simulink model "localization"  (R2025a)
settings: Solver=ode1  StartTime=0.0  StopTime=Inf  FixedStep=0.2  RelTol=1e-3
PostLoadFcn:
  | qlabs_setup
model workspace (MAT data in the model file):
  mainStepSize = Simulink.Parameter
  mainStepSize.Value = Simulink.data.Expression
  mainStepSize.Value.ExpressionString = "qc_get_step_size"
  mainStepSize.Complexity = 'real'
  mainStepSize.Dimensions = -1
  mainStepSize.DataType = 'auto'
  mode = Simulink.Parameter
  mode.Value = 1
  mode.Complexity = 'real'
  mode.Dimensions = [1 1]
  mode.Description = '0 - education speeds via wheel speed commands
    | 1 - education speeds via body speed commands
    | 2 - research speeds via wheel speed commands
    | 3 - research speeds via body speed commands'
  mode.DataType = 'auto'
  realSenseStepSize = Simulink.Parameter
  realSenseStepSize.Value = Simulink.data.Expression
  realSenseStepSize.Value.ExpressionString = "qc_get_step_size*ceil(1/30/qc_get_step_size)"
  realSenseStepSize.Complexity = 'real'
  realSenseStepSize.Dimensions = -1
  realSenseStepSize.DataType = 'auto'
undefined symbols (not defined in the file): Point
libraries: quarc_library x17, simulink x1
settings Model: SimulationMode=external  ExtModeTrigDuration=10000  Creator=mbohra  LastModifiedBy=rdu
settings DebuggingCC: UnderspecifiedInitializationDetection=Classic  MergeDetectMultiDrivingBlocksExec=none
settings ModelReferenceCC: PropagateSignalLabelsOutOfModel=off
settings RTWCC: GPUComputeCapability=3.5

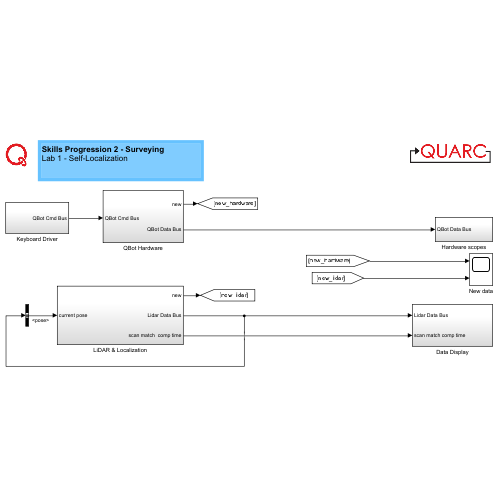
[thumbnail: Simulink's stored preview of the top-level diagram]
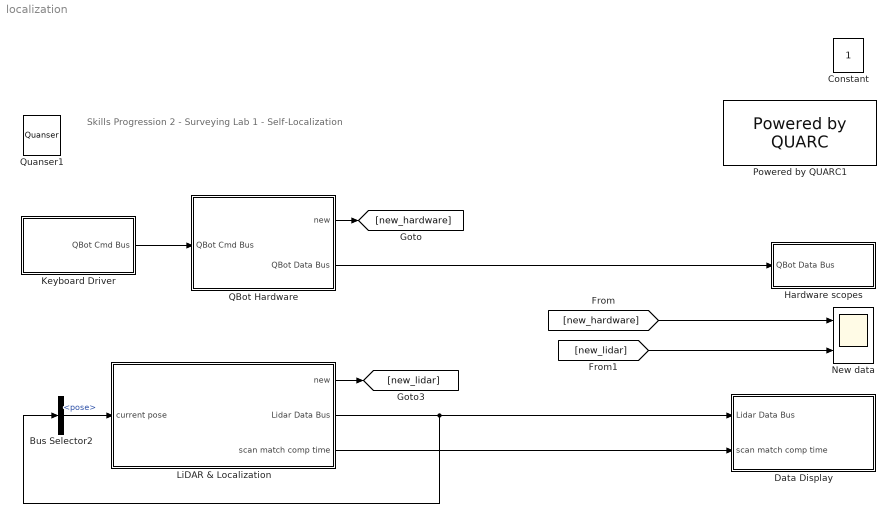
== system localization ==
  note: Skills Progression 2 - Surveying
      | Lab 1 - Self-Localization
  Bus Selector2 : BusSelector  OutputSignals=pose
  Data Display : Subsystem
  Hardware scopes : Subsystem
  Keyboard Driver : Subsystem
  LiDAR & Localization : Subsystem
  New data : Scope  NumInputPorts=2
      settings: Title=Lidar Data New?  ActiveDisplayYMinimum=0.9  ActiveDisplayYMaximum=1.1  DataLoggingVariableName=ScopeData2
  Powered by QUARC1 : quarc_library/Logos/Powered by QUARC
  QBot Hardware : Subsystem
  Quanser1 : quarc_library/Logos/Quanser
  Constant : Constant  IOType=siggen  VectorParams1D=off  SampleTime=1
  wires:
  QBot Hardware/2(QBot Data Bus) -> Hardware scopes/1(QBot Data Bus)
  QBot Hardware/1(new) -> [new_hardware]
  LiDAR & Localization/1(new) -> [new_lidar]
  [new_lidar] -> New data/2
  [new_hardware] -> New data/1
  LiDAR & Localization/2(Lidar Data Bus) -> Data Display/1(Lidar Data Bus), Bus Selector2/1
  Bus Selector2/1 -> LiDAR & Localization/1(current pose)  "<pose>"
  LiDAR & Localization/3(scan match comp time) -> Data Display/2(scan match comp time)
  Keyboard Driver/1(QBot Cmd Bus) -> QBot Hardware/1(QBot Cmd Bus)

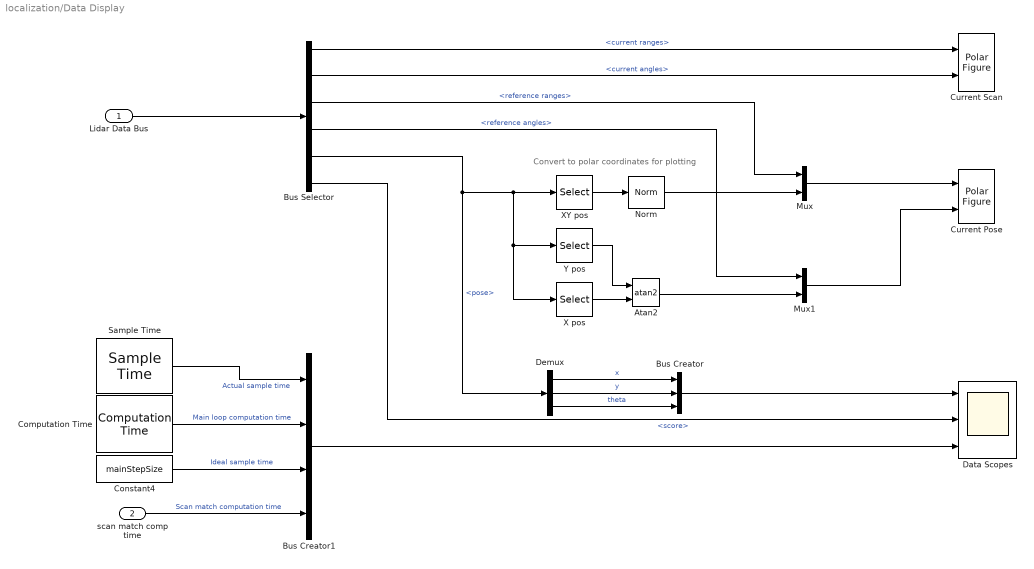
== system localization/Data Display ==
  note: Convert to polar coordinates for plotting
  Lidar Data Bus : Inport
  scan match comp time : Inport  Port=2
  Atan2 : Trigonometry  Operator=atan2
  Bus Creator : BusCreator  Inputs=3
  Bus Creator1 : BusCreator  Inputs=4
  Bus Selector : BusSelector  OutputSignals=current ranges,current angles,reference ranges,reference angles,pose,score
  Computation Time : quarc_library/Sources/Time/Computation Time  sample_time=mainStepSize  use_model=on  use_cpu_time=off
  Constant4 : Constant  Value=mainStepSize
  Current Pose : quarc_library/Sinks/Figures/Polar Figure  figure_mode=Use figure window  figure_tag=figure1  axes_tag=axes1  plot_mode=Time-based  minimum_rho=0  maximum_rho=2  minimum_theta=0  maximum_theta=360  zero_location=right  direction=counterclockwise  buffer_size=2  update_rate=1  sample_time=-1  initial_position="-1516   -95  1081   654"  initial_visibility=off  line1_style=None  line1_width=0.5  line1_color=[1 0 0]  marker1=Point (.)  marker1_size=6  marker1_edge_color=[1 0 0]  marker1_face_color=[1 0 0]  line2_style=Solid line (-)  line2_width=0.5  line2_color=[0.85098 0.32549 0.0980392]  marker2=None  marker2_size=6  marker2_edge_color=[0.85098 0.32549 0.0980392]  marker2_face_color=[0.85098 0.32549 0.0980392]  line3_style=Solid line (-)  line3_width=0.5  line3_color=[0.929412 0.694118 0.12549]  marker3=None  marker3_size=6  marker3_edge_color=[0.929412 0.694118 0.12549]  marker3_face_color=[0.929412 0.694118 0.12549]  line4_style=Solid line (-)  line4_width=0.5  line4_color=[0.494118 0.184314 0.556863]  marker4=None  marker4_size=6  marker4_edge_color=[0.494118 0.184314 0.556863]  marker4_face_color=[0.494118 0.184314 0.556863]  line5_style=Solid line (-)  line5_width=0.5  line5_color=[0.466667 0.67451 0.188235]  marker5=None  marker5_size=6  marker5_edge_color=[0.466667 0.67451 0.188235]  marker5_face_color=[0.466667 0.67451 0.188235]
      settings: SourceProductName=QUARC Targets
  Current Scan : quarc_library/Sinks/Figures/Polar Figure  figure_mode=Use figure window  figure_tag=figure1  axes_tag=axes1  plot_mode=Time-based  minimum_rho=0  maximum_rho=4  minimum_theta=0  maximum_theta=360  zero_location=right  direction=counterclockwise  buffer_size=2  update_rate=1  sample_time=-1  initial_position="370  243  940  693"  initial_visibility=off  line1_style=None  line1_width=0.5  line1_color=[1 0 0]  marker1=Point (.)  marker1_size=6  marker1_edge_color=[1 0 0]  marker1_face_color=[1 0 0]  line2_style=Solid line (-)  line2_width=0.5  line2_color=[0.85098 0.32549 0.0980392]  marker2=None  marker2_size=6  marker2_edge_color=[0.85098 0.32549 0.0980392]  marker2_face_color=[0.85098 0.32549 0.0980392]  line3_style=Solid line (-)  line3_width=0.5  line3_color=[0.929412 0.694118 0.12549]  marker3=None  marker3_size=6  marker3_edge_color=[0.929412 0.694118 0.12549]  marker3_face_color=[0.929412 0.694118 0.12549]  line4_style=Solid line (-)  line4_width=0.5  line4_color=[0.494118 0.184314 0.556863]  marker4=None  marker4_size=6  marker4_edge_color=[0.494118 0.184314 0.556863]  marker4_face_color=[0.494118 0.184314 0.556863]  line5_style=Solid line (-)  line5_width=0.5  line5_color=[0.466667 0.67451 0.188235]  marker5=None  marker5_size=6  marker5_edge_color=[0.466667 0.67451 0.188235]  marker5_face_color=[0.466667 0.67451 0.188235]
      settings: SourceProductName=QUARC Targets
  Data Scopes : Scope  NumInputPorts=3
      settings: ActiveDisplayString=3  Title=Timing  ActiveDisplayYMinimum=-0.051018299999999989  ActiveDisplayYMaximum=0.45916470000000004
  Demux : Demux  Outputs=3
  Mux : Mux  Inputs=2
  Mux1 : Mux  Inputs=2
  Norm : quarc_library/Math Operations/Vectors/Norm
      settings: SourceProductName=QUARC Targets
  Sample Time : quarc_library/Sources/Time/Sample Time  Priority=-99  sample_time=mainStepSize
  X pos : Selector  InputPortWidth=3  IndexOptions=Index vector (dialog)  Indices=[1]  OutputSizes=1
  "XY pos " : Selector  InputPortWidth=3  IndexOptions=Index vector (dialog)  Indices=[1 2]  OutputSizes=1
  Y pos : Selector  InputPortWidth=3  IndexOptions=Index vector (dialog)  Indices=2  OutputSizes=1
  wires:
  Demux/3 -> Bus Creator/3  "theta"
  Demux/2 -> Bus Creator/2  "y"
  Demux/1 -> Bus Creator/1  "x"
  Bus Creator/1 -> Data Scopes/1
  Bus Selector/6 -> Data Scopes/2  "<score>"
  Sample Time/1 -> Bus Creator1/1  "Actual sample time"
  Computation Time/1 -> Bus Creator1/2  "Main loop computation time"
  Constant4/1 -> Bus Creator1/3  "Ideal sample time"
  Bus Creator1/1 -> Data Scopes/3
  scan match comp time/1 -> Bus Creator1/4  "Scan match computation time"
  Bus Selector/2 -> Current Scan/2  "<current angles>"
  Y pos/1 -> Atan2/1
  Bus Selector/3 -> Mux/1  "<reference ranges>"
  Bus Selector/4 -> Mux1/1  "<reference angles>"
  Bus Selector/1 -> Current Scan/1  "<current ranges>"
  Atan2/1 -> Mux1/2
  Bus Selector/5 -> Demux/1, X pos/1, Y pos/1, "XY pos "/1  "<pose>"
  Norm/1 -> Mux/2
  X pos/1 -> Atan2/2
  "XY pos "/1 -> Norm/1
  Lidar Data Bus/1 -> Bus Selector/1
  Mux/1 -> Current Pose/1
  Mux1/1 -> Current Pose/2

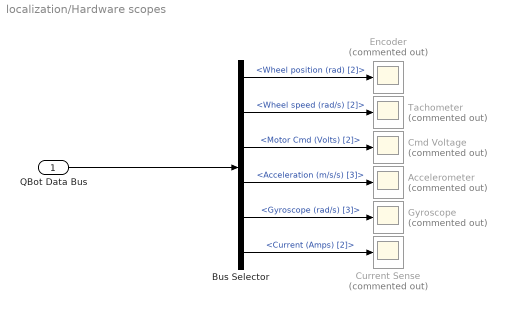
== system localization/Hardware scopes ==
  QBot Data Bus : Inport
  Accelerometer : Scope  Commented=on
      settings: ActiveDisplayYMinimum=-1.32758  ActiveDisplayYMaximum=11.23  DataLoggingVariableName=ScopeData5
  Bus Selector : BusSelector  OutputSignals=Wheel position (rad) [2],Wheel speed (rad/s) [2],Motor Cmd (Volts) [2],Acceleration (m/s/s) [3],Gyroscope (rad/s) [3],Current (Amps) [2]
  Cmd Voltage : Scope  Commented=on
      settings: ActiveDisplayYMinimum=-1  ActiveDisplayYMaximum=1  DataLoggingVariableName=ScopeData4
  Current Sense : Scope  Commented=on
      settings: ActiveDisplayYMinimum=-0.05029  ActiveDisplayYMaximum=0.45265  DataLoggingVariableName=ScopeData7
  Encoder : Scope  Commented=on
      settings: ActiveDisplayYMinimum=-23.46955  ActiveDisplayYMaximum=23.65434  DataLoggingVariableName=ScopeData8
  Gyroscope : Scope  Commented=on
      settings: ActiveDisplayYMinimum=-0.40322  ActiveDisplayYMaximum=1.99912  DataLoggingVariableName=ScopeData6
  Tachometer : Scope  Commented=on
      settings: ActiveDisplayYMinimum=-11.69986  ActiveDisplayYMaximum=11.67552  DataLoggingVariableName=ScopeData3
  wires:
  Bus Selector/2 -> Tachometer/1  "<Wheel speed (rad/s) [2]>"
  Bus Selector/6 -> Current Sense/1  "<Current (Amps) [2]>"
  Bus Selector/3 -> Cmd Voltage/1  "<Motor Cmd (Volts) [2]>"
  Bus Selector/4 -> Accelerometer/1  "<Acceleration (m/s/s) [3]>"
  Bus Selector/5 -> Gyroscope/1  "<Gyroscope (rad/s) [3]>"
  Bus Selector/1 -> Encoder/1  "<Wheel position (rad) [2]>"
  QBot Data Bus/1 -> Bus Selector/1

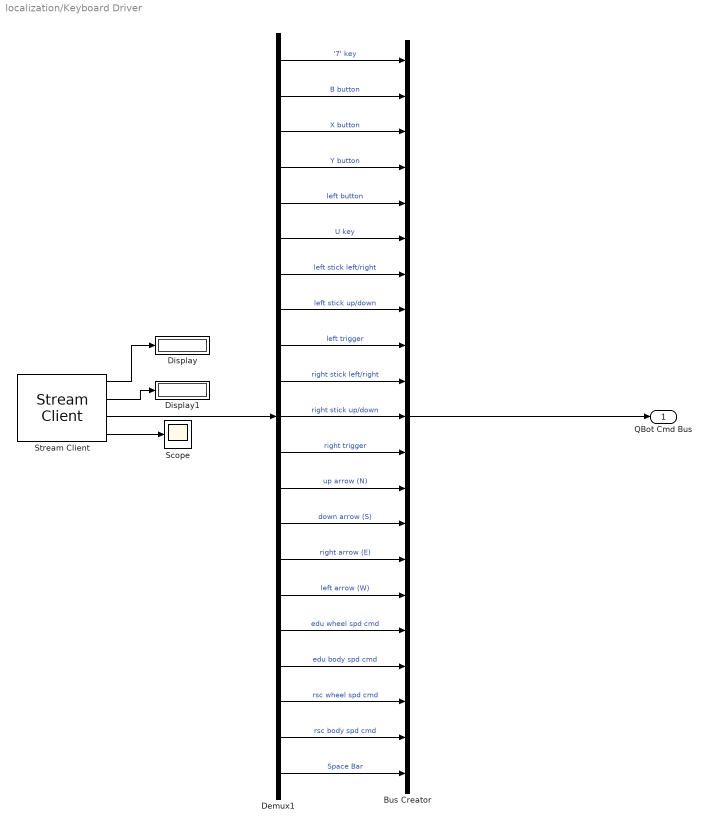
== system localization/Keyboard Driver ==
  Bus Creator : BusCreator  Inputs=21
  Demux1 : Demux  Outputs=[1 1 1 1 1 1 1 1 1 1 1 1 1 1 1 1 2 2 2 2 1]
  Display : Display
  Display1 : Display
  Scope : Scope
      settings: ActiveDisplayYMinimum=-0.125  ActiveDisplayYMaximum=1.125
  Stream Client : quarc_library/Communications/Basic/Stream Client  uri_source=Specify via dialog (do not evaluate)  uri=tcpip://localhost:18889?nagle='off'  send_buffer_size=1460  receive_buffer_size=1460  byte_order=little endian (Intel - LSB first)  optimization=Minimum latency  send_options=Do not send data  receive_options=Receive most recent data  default_value=zeros(25,1)  sample_time=mainStepSize  active=on  implementation=Use blocking I/O in a separate thread  send_fifo_size=1000  receive_fifo_size=1000  send_priority=0  receive_priority=0  send_dimensions=off  receive_dimensions=off  max_dimensions=-1  data_type=Inherited via back propagation  type_expr=BusObject
      settings: AttributesFormatString="\"tcpip://localhost:18889?nagle='off'\""
  QBot Cmd Bus : Outport
  wires:
  Bus Creator/1 -> QBot Cmd Bus/1
  Stream Client/3 -> Demux1/1
  Demux1/1 -> Bus Creator/1  "'7' key"
  Demux1/2 -> Bus Creator/2  "B button"
  Demux1/3 -> Bus Creator/3  "X button"
  Demux1/4 -> Bus Creator/4  "Y button"
  Demux1/5 -> Bus Creator/5  "left button"
  Demux1/6 -> Bus Creator/6  "U key"
  Demux1/7 -> Bus Creator/7  "left stick left/right"
  Demux1/8 -> Bus Creator/8  "left stick up/down"
  Demux1/9 -> Bus Creator/9  "left trigger"
  Demux1/10 -> Bus Creator/10  "right stick left/right"
  Demux1/11 -> Bus Creator/11  "right stick up/down"
  Demux1/12 -> Bus Creator/12  "right trigger"
  Demux1/13 -> Bus Creator/13  "up arrow (N)"
  Demux1/14 -> Bus Creator/14  "down arrow (S)"
  Demux1/15 -> Bus Creator/15  "right arrow (E)"
  Demux1/16 -> Bus Creator/16  "left arrow (W)"
  Demux1/17 -> Bus Creator/17  "edu wheel spd cmd"
  Demux1/18 -> Bus Creator/18  "edu body spd cmd"
  Demux1/19 -> Bus Creator/19  "rsc wheel spd cmd"
  Demux1/20 -> Bus Creator/20  "rsc body spd cmd"
  Demux1/21 -> Bus Creator/21  "Space Bar"
  Stream Client/1 -> Display/1
  Stream Client/2 -> Display1/1
  Stream Client/4 -> Scope/1

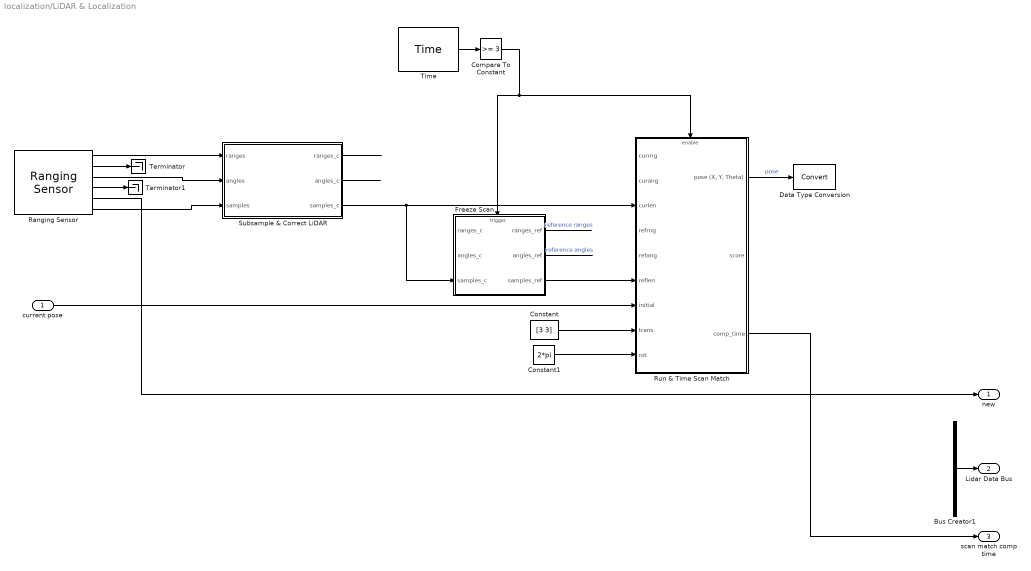
== system localization/LiDAR & Localization ==
  current pose : Inport
  Bus Creator1 : BusCreator  Inputs=6
  Compare To Constant : simulink/Logic and Bit Operations/Compare To Constant  relop=>=  const=3  OutDataTypeStr=boolean
  Constant : Constant  Value=[3 3]
  Constant1 : Constant  Value=2*pi
  Data Type Conversion : DataTypeConversion  SaturateOnIntegerOverflow=off  RndMeth=Floor
  Freeze Scan : Subsystem  TreatAsAtomicUnit=on
  Ranging Sensor : quarc_library/Devices/Third-Party/Sensors/Ranging Sensor  sensor_type=Leishen M10P LIDAR  uri=tcpip://localhost:18918  ranging_distance=Short  timing_budget=0.033  measurement_period=0.0005  output_mode=Fixed-size output  samples_per_revolution=1680  max_distance=0.050  max_angle=5  sample_time=mainStepSize  show_versions=off  active=on
      settings: SourceProductName=QUARC Targets
  "Run & Time Scan Match " : Subsystem
  Subsample & Correct LiDAR : Subsystem
  Terminator : Terminator
  Terminator1 : Terminator
  Time : quarc_library/Sources/Time/Time  time_source=Wall clock  sample_time=mainStepSize
  new : Outport
  Lidar Data Bus : Outport  Port=2
  scan match comp time : Outport  Port=3
  wires:
  Ranging Sensor/5 -> new/1
  Ranging Sensor/2 -> Terminator/1
  Ranging Sensor/4 -> Terminator1/1
  Compare To Constant/1 -> "Run & Time Scan Match "/Enable, Freeze Scan/Trigger
  "Run & Time Scan Match "/1("pose (X, Y, Theta)") -> Data Type Conversion/1  "pose"
  Freeze Scan/3(samples_ref) -> "Run & Time Scan Match "/6(reflen)
  Time/1 -> Compare To Constant/1
  Bus Creator1/1 -> Lidar Data Bus/1
  current pose/1 -> "Run & Time Scan Match "/7(initial)
  Constant/1 -> "Run & Time Scan Match "/8(trans)
  Constant1/1 -> "Run & Time Scan Match "/9(rot)
  "Run & Time Scan Match "/3(comp_time) -> scan match comp time/1
  Ranging Sensor/1 -> Subsample & Correct LiDAR/1(ranges)
  Ranging Sensor/3 -> Subsample & Correct LiDAR/2(angles)
  Ranging Sensor/6 -> Subsample & Correct LiDAR/3(samples)
  ? -> Freeze Scan/1(ranges_c)
  ? -> Freeze Scan/2(angles_c)
  Subsample & Correct LiDAR/3(samples_c) -> Freeze Scan/3(samples_c), "Run & Time Scan Match "/3(curlen)
  Subsample & Correct LiDAR/1(ranges_c) -> ?
  Subsample & Correct LiDAR/2(angles_c) -> ?
  ? -> Bus Creator1/1  "current ranges"
  ? -> Bus Creator1/2  "current angles"
  ? -> Bus Creator1/3  "reference ranges"
  ? -> Bus Creator1/4  "reference angles"
  ? -> Bus Creator1/5  "pose"
  ? -> Bus Creator1/6  "score"
  Freeze Scan/1(ranges_ref) -> ?  "reference ranges"
  Freeze Scan/2(angles_ref) -> ?  "reference angles"

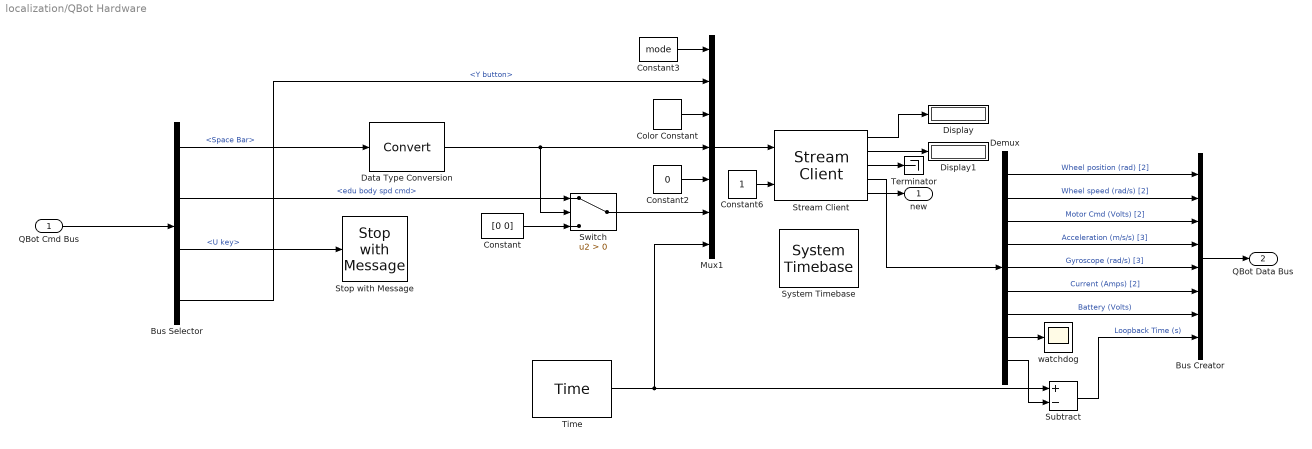
== system localization/QBot Hardware ==
  QBot Cmd Bus : Inport
  Bus Creator : BusCreator  Inputs=8
  Bus Selector : BusSelector  OutputSignals=Space Bar,edu body spd cmd,U key,Y button
  Color Constant : quarc_library/Sources/Signals/Color Constant  color=[1 0 1]
      settings: SourceProductName=QUARC Targets
  Constant : Constant  Value=[0 0]
  Constant2 : Constant  Value=0
  Constant3 : Constant  Value=mode
  Constant6 : Constant
  Data Type Conversion : DataTypeConversion  SaturateOnIntegerOverflow=off  RndMeth=Floor
  Demux : Demux  Outputs=[2 2 2 3 3 2 1 1 1]
  Display : Display
  Display1 : Display
  Mux1 : Mux  Inputs=7
  Stop with Message : quarc_library/Sinks/Error Handling/Stop with Message  message_type=Fixed error message  message_icon=Information  message=Operator: Emergency Stop
  Stream Client : quarc_library/Communications/Basic/Stream Client  uri_source=Specify via dialog (do not evaluate)  uri=tcpip://localhost:18888  send_buffer_size=1460  receive_buffer_size=1460  byte_order=little endian (Intel - LSB first)  optimization=Minimum latency  send_options=Send most recent data  receive_options=Receive most recent data  default_value=zeros(17,1)  sample_time=mainStepSize  active=on  implementation=Use blocking I/O in a separate thread  send_fifo_size=1000  receive_fifo_size=1000  send_priority=0  receive_priority=0  send_dimensions=off  receive_dimensions=off  max_dimensions=-1  data_type=Inherited via back propagation  type_expr=BusObject
      settings: AttributesFormatString="\"tcpip://localhost:18888\""
  Subtract : Sum  Inputs=+-
  Switch : Switch  Criteria=u2 > Threshold  SaturateOnIntegerOverflow=off  InputSameDT=off
  System Timebase : quarc_library/Advanced/Timing/System Timebase  stop_on_overrun=off
      settings: SourceProductName=QUARC Targets
  Terminator : Terminator
  Time : quarc_library/Sources/Time/Time  time_source=Wall clock  sample_time=qc_get_step_size
  watchdog : Scope
  new : Outport
  QBot Data Bus : Outport  Port=2
  wires:
  Demux/2 -> Bus Creator/2  "Wheel speed (rad/s) [2]"
  Constant3/1 -> Mux1/1
  Stream Client/3 -> Terminator/1
  Bus Selector/2 -> Switch/1  "<edu body spd cmd>"
  Stream Client/1 -> Display/1
  Constant6/1 -> Stream Client/2
  Stream Client/2 -> Display1/1
  Color Constant/1 -> Mux1/3
  Demux/3 -> Bus Creator/3  "Motor Cmd (Volts) [2]"
  Mux1/1 -> Stream Client/1
  Stream Client/4 -> Demux/1
  Demux/1 -> Bus Creator/1  "Wheel position (rad) [2]"
  Stream Client/5 -> new/1
  Demux/7 -> Bus Creator/7  "Battery (Volts)"
  Demux/5 -> Bus Creator/5  "Gyroscope (rad/s) [3]"
  Demux/6 -> Bus Creator/6  "Current (Amps) [2]"
  Demux/9 -> Subtract/2
  Constant2/1 -> Mux1/5
  Demux/4 -> Bus Creator/4  "Acceleration (m/s/s) [3]"
  Time/1 -> Mux1/7, Subtract/1
  Bus Creator/1 -> QBot Data Bus/1
  Subtract/1 -> Bus Creator/8  "Loopback Time (s)"
  Demux/8 -> watchdog/1
  Switch/1 -> Mux1/6
  Constant/1 -> Switch/3
  QBot Cmd Bus/1 -> Bus Selector/1
  Bus Selector/3 -> Stop with Message/1  "<U key>"
  Bus Selector/1 -> Data Type Conversion/1  "<Space Bar>"
  Data Type Conversion/1 -> Mux1/4, Switch/2
  Bus Selector/4 -> Mux1/2  "<Y button>"

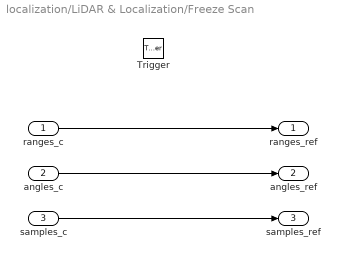
== system localization/LiDAR & Localization/Freeze Scan ==
  ranges_c : Inport
  angles_c : Inport  Port=2
  samples_c : Inport  Port=3
  Trigger : TriggerPort  VariantControl=(inherit)  InitialTriggerSignalState=zero
  ranges_ref : Outport
  angles_ref : Outport  Port=2
  samples_ref : Outport  Port=3
  wires:
  ranges_c/1 -> ranges_ref/1
  angles_c/1 -> angles_ref/1
  samples_c/1 -> samples_ref/1

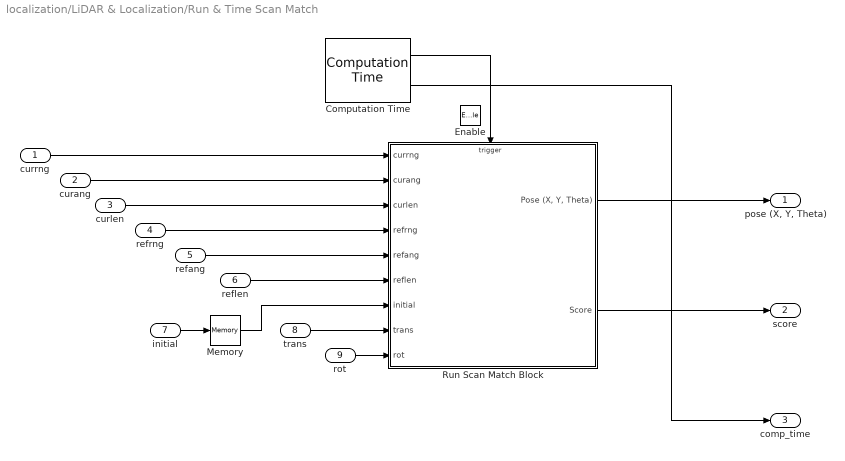
== system localization/LiDAR & Localization/Run & Time Scan Match  ==
  currng : Inport
  curang : Inport  Port=2
  curlen : Inport  Port=3
  refrng : Inport  Port=4
  refang : Inport  Port=5
  reflen : Inport  Port=6
  initial : Inport  Port=7
  trans : Inport  Port=8
  rot : Inport  Port=9
  Enable : EnablePort
  Computation Time : quarc_library/Sources/Time/Computation Time  sample_time=mainStepSize  use_model=off  use_cpu_time=off
  Memory : Memory  InheritSampleTime=on
  "Run Scan Match Block " : Subsystem  TreatAsAtomicUnit=on
  "pose (X, Y, Theta)" : Outport
  score : Outport  Port=2
  comp_time : Outport  Port=3
  wires:
  currng/1 -> "Run Scan Match Block "/1(currng)
  curang/1 -> "Run Scan Match Block "/2(curang)
  curlen/1 -> "Run Scan Match Block "/3(curlen)
  refrng/1 -> "Run Scan Match Block "/4(refrng)
  refang/1 -> "Run Scan Match Block "/5(refang)
  reflen/1 -> "Run Scan Match Block "/6(reflen)
  initial/1 -> Memory/1
  trans/1 -> "Run Scan Match Block "/8(trans)
  rot/1 -> "Run Scan Match Block "/9(rot)
  Computation Time/1 -> "Run Scan Match Block "/Trigger
  Computation Time/2 -> comp_time/1
  "Run Scan Match Block "/1("Pose (X, Y, Theta)") -> "pose (X, Y, Theta)"/1
  "Run Scan Match Block "/2(Score) -> score/1
  Memory/1 -> "Run Scan Match Block "/7(initial)

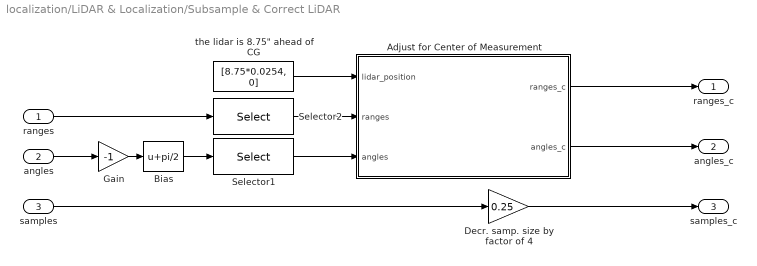
== system localization/LiDAR & Localization/Subsample & Correct LiDAR ==
  ranges : Inport
  angles : Inport  Port=2
  samples : Inport  Port=3
  Adjust for Center of Measurement : MATLAB Function  TreatAsAtomicUnit=on  SystemSampleTime=mainStepSize
  Bias : Bias  Bias=pi/2  SaturateOnIntegerOverflow=off
  "Decr. samp. size by factor of 4 " : Gain  Gain=0.25  OutDataTypeStr=int32
  Gain : Gain  Gain=-1
  Selector1 : Selector  InputPortWidth=1680  IndexOptions=Index vector (dialog)  Indices=[1:4:1677]  OutputSizes=1
  Selector2 : Selector  InputPortWidth=1680  IndexOptions=Index vector (dialog)  Indices=[1:4:1677]  OutputSizes=1
  "the lidar is 8.75\" ahead of CG" : Constant  Value=[8.75*0.0254, 0]  SampleTime=mainStepSize
  ranges_c : Outport
  angles_c : Outport  Port=2
  samples_c : Outport  Port=3
  wires:
  "the lidar is 8.75\" ahead of CG"/1 -> Adjust for Center of Measurement/1(lidar_position)
  Selector2/1 -> Adjust for Center of Measurement/2(ranges)
  angles/1 -> Gain/1
  Bias/1 -> Selector1/1
  samples/1 -> "Decr. samp. size by factor of 4 "/1
  Gain/1 -> Bias/1
  ranges/1 -> Selector2/1
  Selector1/1 -> Adjust for Center of Measurement/3(angles)
  Adjust for Center of Measurement/1(ranges_c) -> ranges_c/1
  Adjust for Center of Measurement/2(angles_c) -> angles_c/1
  "Decr. samp. size by factor of 4 "/1 -> samples_c/1

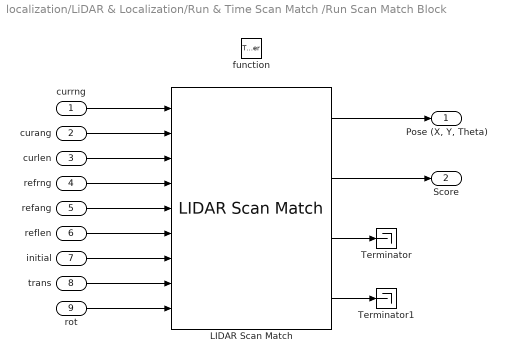
== system localization/LiDAR & Localization/Run & Time Scan Match /Run Scan Match Block  ==
  currng : Inport
  curang : Inport  Port=2
  curlen : Inport  Port=3
  refrng : Inport  Port=4
  refang : Inport  Port=5
  reflen : Inport  Port=6
  initial : Inport  Port=7
  trans : Inport  Port=8
  rot : Inport  Port=9
  function : TriggerPort  TriggerType=function-call  VariantControl=(inherit)
  LIDAR Scan Match : quarc_library/Image Processing/Generic/LIDAR Scan Match  mode=Fixed input with size  resolution=40  max_range=5  use_initial_pose=on
      settings: SourceProductName=QUARC Targets
  Terminator : Terminator
  Terminator1 : Terminator
  "Pose (X, Y, Theta)" : Outport
  Score : Outport  Port=2
  wires:
  rot/1 -> LIDAR Scan Match/9
  LIDAR Scan Match/2 -> Score/1
  trans/1 -> LIDAR Scan Match/8
  initial/1 -> LIDAR Scan Match/7
  refang/1 -> LIDAR Scan Match/5
  reflen/1 -> LIDAR Scan Match/6
  LIDAR Scan Match/4 -> Terminator1/1
  currng/1 -> LIDAR Scan Match/1
  LIDAR Scan Match/1 -> "Pose (X, Y, Theta)"/1
  curang/1 -> LIDAR Scan Match/2
  LIDAR Scan Match/3 -> Terminator/1
  curlen/1 -> LIDAR Scan Match/3
  refrng/1 -> LIDAR Scan Match/4

== matlab function localization/LiDAR & Localization/Subsample & Correct LiDAR/Adjust for Center of Measurement ==
  data: lidar_position input; ranges input; ranges_c output; angles input; angles_c output
function [ranges_c,angles_c] = correct_lidar(lidar_position, ranges,angles)

% Convert lidar data from polar into cartesian, and add lidar position
% Then Convert back into polar coordinates
%-------Replace the following line with your code---------%
ranges_c = ranges;
angles_c = angles./angles;
%---------------------------------------------------------%

end
